simulink model "FOC"  (R2021b)
settings: Solver=ode45  StartTime=0.0  StopTime=1  MaxStep=1e-6  RelTol=1e-3
undefined symbols (not defined in the file): F, Flux, J, Ki_cd, Ki_cq, Ki_w, Kp_cd, Kp_cq, Kp_w, Ld, Lq, Np, Rs, Tf, Tmax, Tn, Ts, Udc, wn
libraries: slpidlib x3, spsUniversalBridgeLib x2, spsPermanentMagnetSynchronousMachineLib x1, spsSeriesRLCBranchLib x1, spsOnDelayLib x1, simulink x1, spsThreePhaseSourceLib x1, spsVoltageMeasurementLib x1, spspowerguiLib x1
settings Model: SimulationMode=accelerator  Creator=LFL  LastModifiedBy=Jiaxin Qian
settings SolverCC: AlgebraicLoopSolver=TrustRegion
settings DataIOCC: ReturnWorkspaceOutputs=off
settings DebuggingCC: SFMachineParentedDataDiag=warning  ArithmeticOperatorsInVariantConditions=warning
settings SFSimCC: SimUseLocalCustomCode=off  CustomCodeUndefinedFunction=UseInterfaceOnly
settings RTWCC: RTWUseLocalCustomCode=off

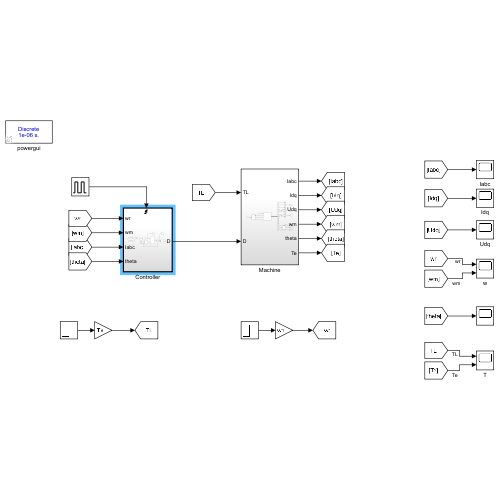
[thumbnail: Simulink's stored preview of the top-level diagram]
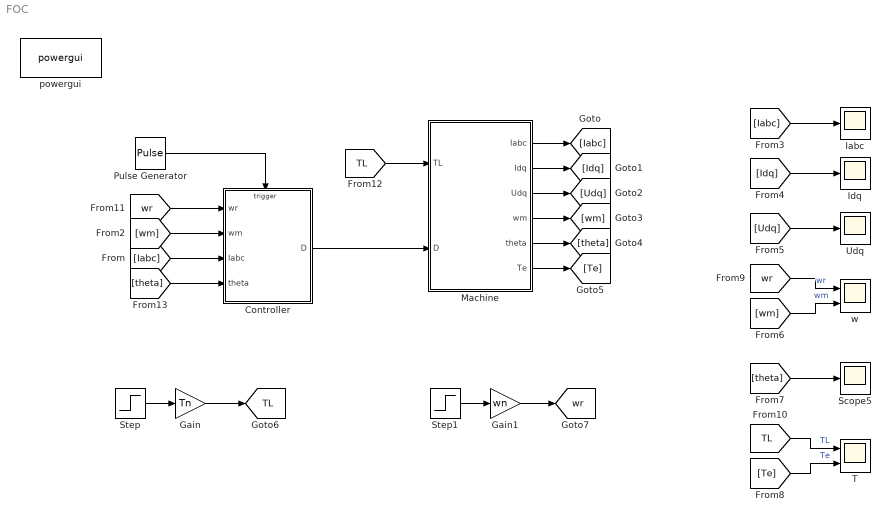
== system FOC ==
  Controller : Subsystem  TreatAsAtomicUnit=on
  Gain : Gain  Gain=Tn
  Gain1 : Gain  Gain=wn
  Iabc : Scope
  Idq : Scope
  Machine : Subsystem
  Pulse Generator : DiscretePulseGenerator  PulseType=Time based  Period=Ts  PulseWidth=50
  Scope5 : Scope
  Step : Step  Time=0.5  SampleTime=0
  Step1 : Step  Time=0  SampleTime=0
  T : Scope  NumInputPorts=2
  Udq : Scope
  powergui : spspowerguiLib/powergui  Priority=1  SimulationMode=Discrete  SampleTime=1e-6  frequency=60  Iterations=50  frequencyindice=0  Pbase=100e6  ErrMax=1e-4  UnitsV=kV  UnitsW=MW  buscounter=0  FunctionMessages=off  echomessages=off  EnableUseOfTLC=off  CurrentSourceSwitches=off  DisableSnubberDevices=off  DisableRonSwitches=off  DisableVfSwitches=off  DisplayEquations=off  AutomaticDiscreteSolvers=off  SolverType=Tustin/Backward Euler (TBE)  Interpol=off  ExternalGateDelay=off  methode=off  Ts=100  x0status=blocks  SPID=on  SwTol=0  HookPort=off  NonlinearTolerance=1e-4  nMaxIteration=100  ContinueOnMaxIteration=off  RestoreLinks=warning  ResistiveCurrentMeasurement=off  Frange=[0:2:500]  Ylog=off  Xlog=on  ShowGrid=off  save=off  variable=ZData  structure=0  ZoomFFT=off  StartTime=0.0  cycles=1  DisplayStyle=1  fundamental=60  FreqAxis=off  MaxFrequency=1000  frequencyindicesteady=1  RmsSteady=1  display=off
  w : Scope  NumInputPorts=2
  tag scope: TL=global, wr=global
  wires:
  Controller/1(D) -> Machine/2(D)
  Pulse Generator/1 -> Controller/Trigger
  Machine/1(Iabc) -> [Iabc]
  Machine/2(Idq) -> [Idq]
  Machine/3(Udq) -> [Udq]
  Machine/4(wm) -> [wm]
  Machine/5(theta) -> [theta]
  Machine/6(Te) -> [Te]
  [Iabc] -> Controller/3(Iabc)
  [wm] -> Controller/2(wm)
  [Iabc] -> Iabc/1
  [Udq] -> Udq/1
  [wm] -> w/2  "wm"
  [wr] -> w/1  "wr"
  [TL] -> T/1  "TL"
  [Te] -> T/2  "Te"
  [theta] -> Scope5/1
  [Idq] -> Idq/1
  [wr] -> Controller/1(wr)
  [TL] -> Machine/1(TL)
  [theta] -> Controller/4(theta)
  Step/1 -> Gain/1
  Gain/1 -> [TL]
  Step1/1 -> Gain1/1
  Gain1/1 -> [wr]

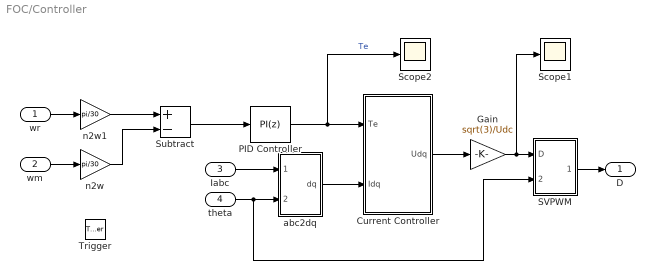
== system FOC/Controller ==
  wr : Inport
  wm : Inport  Port=2
  Iabc : Inport  Port=3
  theta : Inport  Port=4
  Trigger : TriggerPort  VariantControl=Variant
  Current Controller : Subsystem
  Gain : Gain  Gain=sqrt(3)/Udc
  PID Controller : slpidlib/PID Controller  Controller=PI  Form=Parallel  TimeDomain=Discrete-time  UseExternalTs=off  SampleTime=-1  IntegratorMethod=Forward Euler  FilterMethod=Forward Euler  ControllerParametersSource=internal  P=Kp_w  I=Ki_w  D=0  UseFilter=on  N=100  TunerSelectOption=Transfer Function Based (PID Tuner App)  InitialConditionSource=internal  InitialConditionForIntegrator=0  InitialConditionForFilter=0  DifferentiatorICPrevScaledInput=0  ExternalReset=none  TrackingMode=off  Kt=1  LimitOutput=on  SatLimitsSource=internal  UpperSaturationLimit=Tmax  LowerSaturationLimit=-Tmax  LinearizeAsGain=on  AntiWindupMode=clamping  Kb=1  POutMin=[]  POutMax=[]  IOutMin=[]  IOutMax=[]  DOutMin=[]  DOutMax=[]  NOutMin=[]  NOutMax=[]  SumOutMin=[]  SumOutMax=[]  SaturationOutMin=[]  SaturationOutMax=[]  PParamMin=[]  PParamMax=[]  IParamMin=[]  IParamMax=[]  DParamMin=[]  DParamMax=[]  NParamMin=[]  NParamMax=[]  KbParamMin=[]  KbParamMax=[]  KtParamMin=[]  KtParamMax=[]  KbOutMin=[]  KbOutMax=[]  KtOutMin=[]  KtOutMax=[]  IntegratorOutMin=[]  IntegratorOutMax=[]  FilterOutMin=[]  FilterOutMax=[]  SumI1OutMin=[]  SumI1OutMax=[]  SumI2OutMin=[]  SumI2OutMax=[]  SumI3OutMin=[]  SumI3OutMax=[]  SumI4OutMin=[]  SumI4OutMax=[]  SumDOutMin=[]  SumDOutMax=[]  DifferentiatorOutMin=[]  DifferentiatorOutMax=[]  FilterDiffOutCoefMin=[]  FilterDiffOutCoefMax=[]  ReciprocalOutMin=[]  ReciprocalOutMax=[]  SumDenOutMin=[]  SumDenOutMax=[]  SumNumOutMin=[]  SumNumOutMax=[]  DivideOutMin=[]  DivideOutMax=[]  UdiffTsProdOutMin=[]  UdiffTsProdOutMax=[]  NTsProdOutMin=[]  NTsProdOutMax=[]  UintegralTsProdOutMin=[]  UintegralTsProdOutMax=[]  UngainTsProdOutMin=[]  UngainTsProdOutMax=[]  IntegratorContinuousStateAttributes=''  IntegratorStateMustResolveToSignalObject=off  IntegratorRTWStateStorageClass=Auto  FilterContinuousStateAttributes=''  FilterStateMustResolveToSignalObject=off  FilterRTWStateStorageClass=Auto  ParallelPVariant=InternalParameters  IdealPVariant=Disabled  IVariant=InternalParameters  DVariant=Disabled  IntegratorVariant=Discrete  SatVariant=Enabled  AWVariant=DiscClampingParallel  PCopyVariant=Disabled  TRVariant=Disabled  FdbkBlocksVariant=Forward  IdealPFdbkVariant=Disabled  SatFdbkVariant=Disabled  DerivativeFilterVariant=Disabled  NVariant=Disabled  NCopyVariant=Disabled_SignalSpec  FilterICVariant=Disabled  IntegratorICVariant=InternalICs  ExternalResetVariant=Disabled  TRSumVariant=Passthrough  SumFdbkVariant=Disabled  SumVariant=Sum_PI  TsampFilterVariant=InternalTs  TsampNgainVariant=Passthrough  TsampIntegralVariant=Passthrough  ExternalSaturationOutDataTypeStr=Inherit: Same as second input
  SVPWM : Subsystem
  Scope1 : Scope
  Scope2 : Scope
  Subtract : Sum  Inputs=+-
  abc2dq : Subsystem
  n2w : Gain  Gain=pi/30
  n2w1 : Gain  Gain=pi/30
  D : Outport  VectorParamsAs1DForOutWhenUnconnected=off
  wires:
  wr/1 -> n2w1/1
  wm/1 -> n2w/1
  Subtract/1 -> PID Controller/1
  PID Controller/1 -> Scope2/1, Current Controller/1(Te)  "Te"
  Current Controller/1(Udq) -> Gain/1
  Gain/1 -> SVPWM/1(D), Scope1/1
  n2w/1 -> Subtract/2
  n2w1/1 -> Subtract/1
  abc2dq/1(dq) -> Current Controller/2(Idq)
  Iabc/1 -> abc2dq/1(abc)
  SVPWM/1(Dabc) -> D/1
  theta/1 -> SVPWM/2(theta), abc2dq/2(theta)

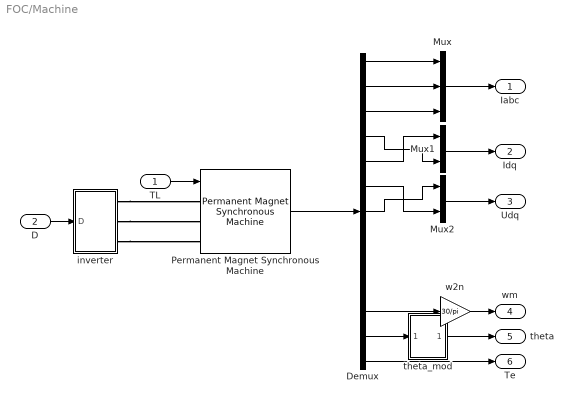
== system FOC/Machine ==
  TL : Inport
  D : Inport  Port=2
  Demux : Demux  Outputs=13
  Mux : Mux  Inputs=3
  Mux1 : Mux  Inputs=2
  Mux2 : Mux  Inputs=2
  Permanent Magnet Synchronous Machine : spsPermanentMagnetSynchronousMachineLib/Permanent Magnet Synchronous Machine  NbPhases=3  FluxDistribution=Sinusoidal  RotorType=Salient-pole  MechanicalLoad=Torque Tm  PresetModel=No  ShowDetailedParameters=on  MeasurementBus=off  Resistance=Rs  Inductance=8.5e-3  dqInductances=[Ld,Lq]  La=0.000395  MachineConstant=Flux linkage established by magnets (V.s)  Flux=Flux  VoltageCst=366.2061  TorqueCst=3.0285  Flat=120  Mechanical=[J F Np Tf]  PolePairs=4  InitialConditions=[0,0, 0,0]  InitialConditions5ph=[0 0 0 0 0 0]  RefAngle=Aligned with phase A axis (original Park)  IterativeDiscreteModel=Trapezoidal non iterative  TsBlock=-1  TsPowergui=0
  inverter : Subsystem
  theta_mod : Subsystem
  w2n : Gain  Gain=30/pi
  Iabc : Outport  VectorParamsAs1DForOutWhenUnconnected=off
  Idq : Outport  Port=2  VectorParamsAs1DForOutWhenUnconnected=off
  Udq : Outport  Port=3  VectorParamsAs1DForOutWhenUnconnected=off
  wm : Outport  Port=4  VectorParamsAs1DForOutWhenUnconnected=off
  theta : Outport  Port=5  VectorParamsAs1DForOutWhenUnconnected=off
  Te : Outport  Port=6  VectorParamsAs1DForOutWhenUnconnected=off
  wires:
  Permanent Magnet Synchronous Machine/1 -> Demux/1
  Demux/1 -> Mux/1
  Demux/2 -> Mux/2
  Demux/3 -> Mux/3
  Mux/1 -> Iabc/1
  Mux1/1 -> Idq/1
  Mux2/1 -> Udq/1
  Demux/11 -> w2n/1
  Demux/12 -> theta_mod/1(In1)
  Demux/13 -> Te/1
  TL/1 -> Permanent Magnet Synchronous Machine/1
  Demux/5 -> Mux1/1
  Demux/4 -> Mux1/2
  Demux/6 -> Mux2/2
  Demux/7 -> Mux2/1
  theta_mod/1(Out1) -> theta/1
  w2n/1 -> wm/1
  D/1 -> inverter/1(D)
  connections:
  inverter/RConn1 -- Permanent Magnet Synchronous Machine/LConn1
  inverter/RConn2 -- Permanent Magnet Synchronous Machine/LConn2
  inverter/RConn3 -- Permanent Magnet Synchronous Machine/LConn3

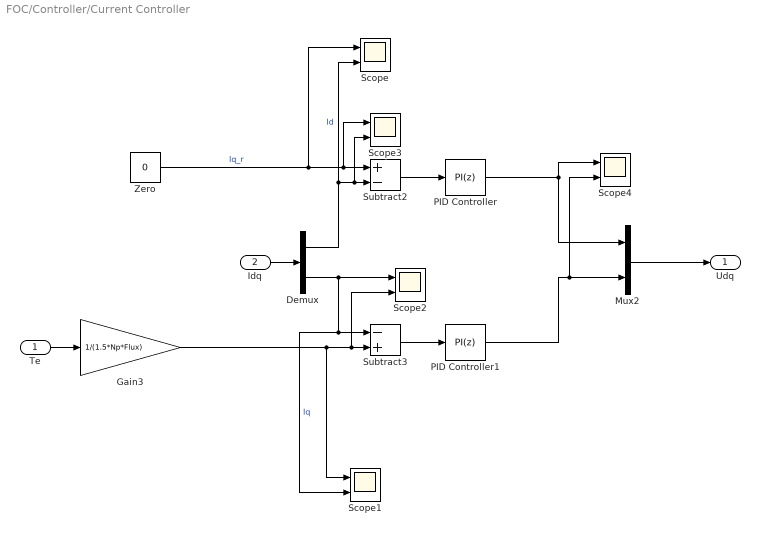
== system FOC/Controller/Current Controller ==
  Te : Inport
  Idq : Inport  Port=2
  Demux : Demux  Outputs=2
  Gain3 : Gain  Gain=1/(1.5*Np*Flux)
  Mux2 : Mux  Inputs=2
  PID Controller : slpidlib/PID Controller  Controller=PI  Form=Parallel  TimeDomain=Discrete-time  UseExternalTs=off  SampleTime=-1  IntegratorMethod=Forward Euler  FilterMethod=Forward Euler  ControllerParametersSource=internal  P=Kp_cd  I=Ki_cd  D=0  UseFilter=on  N=100  TunerSelectOption=Transfer Function Based (PID Tuner App)  InitialConditionSource=internal  InitialConditionForIntegrator=0  InitialConditionForFilter=0  DifferentiatorICPrevScaledInput=0  ExternalReset=none  TrackingMode=off  Kt=1  LimitOutput=off  SatLimitsSource=internal  UpperSaturationLimit=inf  LowerSaturationLimit=-inf  LinearizeAsGain=on  AntiWindupMode=none  Kb=1  POutMin=[]  POutMax=[]  IOutMin=[]  IOutMax=[]  DOutMin=[]  DOutMax=[]  NOutMin=[]  NOutMax=[]  SumOutMin=[]  SumOutMax=[]  SaturationOutMin=[]  SaturationOutMax=[]  PParamMin=[]  PParamMax=[]  IParamMin=[]  IParamMax=[]  DParamMin=[]  DParamMax=[]  NParamMin=[]  NParamMax=[]  KbParamMin=[]  KbParamMax=[]  KtParamMin=[]  KtParamMax=[]  KbOutMin=[]  KbOutMax=[]  KtOutMin=[]  KtOutMax=[]  IntegratorOutMin=[]  IntegratorOutMax=[]  FilterOutMin=[]  FilterOutMax=[]  SumI1OutMin=[]  SumI1OutMax=[]  SumI2OutMin=[]  SumI2OutMax=[]  SumI3OutMin=[]  SumI3OutMax=[]  SumI4OutMin=[]  SumI4OutMax=[]  SumDOutMin=[]  SumDOutMax=[]  DifferentiatorOutMin=[]  DifferentiatorOutMax=[]  FilterDiffOutCoefMin=[]  FilterDiffOutCoefMax=[]  ReciprocalOutMin=[]  ReciprocalOutMax=[]  SumDenOutMin=[]  SumDenOutMax=[]  SumNumOutMin=[]  SumNumOutMax=[]  DivideOutMin=[]  DivideOutMax=[]  UdiffTsProdOutMin=[]  UdiffTsProdOutMax=[]  NTsProdOutMin=[]  NTsProdOutMax=[]  UintegralTsProdOutMin=[]  UintegralTsProdOutMax=[]  UngainTsProdOutMin=[]  UngainTsProdOutMax=[]  IntegratorContinuousStateAttributes=''  IntegratorStateMustResolveToSignalObject=off  IntegratorRTWStateStorageClass=Auto  FilterContinuousStateAttributes=''  FilterStateMustResolveToSignalObject=off  FilterRTWStateStorageClass=Auto  ParallelPVariant=InternalParameters  IdealPVariant=Disabled  IVariant=InternalParameters  DVariant=Disabled  IntegratorVariant=Discrete  SatVariant=Disabled  AWVariant=Passthrough  PCopyVariant=Disabled  TRVariant=Disabled  FdbkBlocksVariant=Forward  IdealPFdbkVariant=Disabled  SatFdbkVariant=Disabled  DerivativeFilterVariant=Disabled  NVariant=Disabled  NCopyVariant=Disabled_SignalSpec  FilterICVariant=Disabled  IntegratorICVariant=InternalICs  ExternalResetVariant=Disabled  TRSumVariant=Passthrough  SumFdbkVariant=Disabled  SumVariant=Sum_PI  TsampFilterVariant=InternalTs  TsampNgainVariant=Passthrough  TsampIntegralVariant=Passthrough  ExternalSaturationOutDataTypeStr=Inherit: Same as second input
  PID Controller1 : slpidlib/PID Controller  Controller=PI  Form=Parallel  TimeDomain=Discrete-time  UseExternalTs=off  SampleTime=-1  IntegratorMethod=Forward Euler  FilterMethod=Forward Euler  ControllerParametersSource=internal  P=Kp_cq  I=Ki_cq  D=0  UseFilter=on  N=100  TunerSelectOption=Transfer Function Based (PID Tuner App)  InitialConditionSource=internal  InitialConditionForIntegrator=0  InitialConditionForFilter=0  DifferentiatorICPrevScaledInput=0  ExternalReset=none  TrackingMode=off  Kt=1  LimitOutput=off  SatLimitsSource=internal  UpperSaturationLimit=inf  LowerSaturationLimit=-inf  LinearizeAsGain=on  AntiWindupMode=none  Kb=1  POutMin=[]  POutMax=[]  IOutMin=[]  IOutMax=[]  DOutMin=[]  DOutMax=[]  NOutMin=[]  NOutMax=[]  SumOutMin=[]  SumOutMax=[]  SaturationOutMin=[]  SaturationOutMax=[]  PParamMin=[]  PParamMax=[]  IParamMin=[]  IParamMax=[]  DParamMin=[]  DParamMax=[]  NParamMin=[]  NParamMax=[]  KbParamMin=[]  KbParamMax=[]  KtParamMin=[]  KtParamMax=[]  KbOutMin=[]  KbOutMax=[]  KtOutMin=[]  KtOutMax=[]  IntegratorOutMin=[]  IntegratorOutMax=[]  FilterOutMin=[]  FilterOutMax=[]  SumI1OutMin=[]  SumI1OutMax=[]  SumI2OutMin=[]  SumI2OutMax=[]  SumI3OutMin=[]  SumI3OutMax=[]  SumI4OutMin=[]  SumI4OutMax=[]  SumDOutMin=[]  SumDOutMax=[]  DifferentiatorOutMin=[]  DifferentiatorOutMax=[]  FilterDiffOutCoefMin=[]  FilterDiffOutCoefMax=[]  ReciprocalOutMin=[]  ReciprocalOutMax=[]  SumDenOutMin=[]  SumDenOutMax=[]  SumNumOutMin=[]  SumNumOutMax=[]  DivideOutMin=[]  DivideOutMax=[]  UdiffTsProdOutMin=[]  UdiffTsProdOutMax=[]  NTsProdOutMin=[]  NTsProdOutMax=[]  UintegralTsProdOutMin=[]  UintegralTsProdOutMax=[]  UngainTsProdOutMin=[]  UngainTsProdOutMax=[]  IntegratorContinuousStateAttributes=''  IntegratorStateMustResolveToSignalObject=off  IntegratorRTWStateStorageClass=Auto  FilterContinuousStateAttributes=''  FilterStateMustResolveToSignalObject=off  FilterRTWStateStorageClass=Auto  ParallelPVariant=InternalParameters  IdealPVariant=Disabled  IVariant=InternalParameters  DVariant=Disabled  IntegratorVariant=Discrete  SatVariant=Disabled  AWVariant=Passthrough  PCopyVariant=Disabled  TRVariant=Disabled  FdbkBlocksVariant=Forward  IdealPFdbkVariant=Disabled  SatFdbkVariant=Disabled  DerivativeFilterVariant=Disabled  NVariant=Disabled  NCopyVariant=Disabled_SignalSpec  FilterICVariant=Disabled  IntegratorICVariant=InternalICs  ExternalResetVariant=Disabled  TRSumVariant=Passthrough  SumFdbkVariant=Disabled  SumVariant=Sum_PI  TsampFilterVariant=InternalTs  TsampNgainVariant=Passthrough  TsampIntegralVariant=Passthrough  ExternalSaturationOutDataTypeStr=Inherit: Same as second input
  Scope{,1..4} (5 alike) : Scope  NumInputPorts=2
  Subtract2 : Sum  Inputs=+-
  Subtract3 : Sum  Inputs=-+
  Zero : Constant  Value=0
  Udq : Outport  VectorParamsAs1DForOutWhenUnconnected=off
  wires:
  Mux2/1 -> Udq/1
  Idq/1 -> Demux/1
  Demux/1 -> Scope/2, Scope3/2, Subtract2/2  "Id"
  Demux/2 -> Scope2/1, Scope1/2, Subtract3/1  "Iq"
  Subtract2/1 -> PID Controller/1
  Subtract3/1 -> PID Controller1/1
  Zero/1 -> Scope3/1, Subtract2/1, Scope/1  "Iq_r"
  Te/1 -> Gain3/1
  Gain3/1 -> Scope2/2, Subtract3/2, Scope1/1
  PID Controller/1 -> Scope4/1, Mux2/1
  PID Controller1/1 -> Scope4/2, Mux2/2

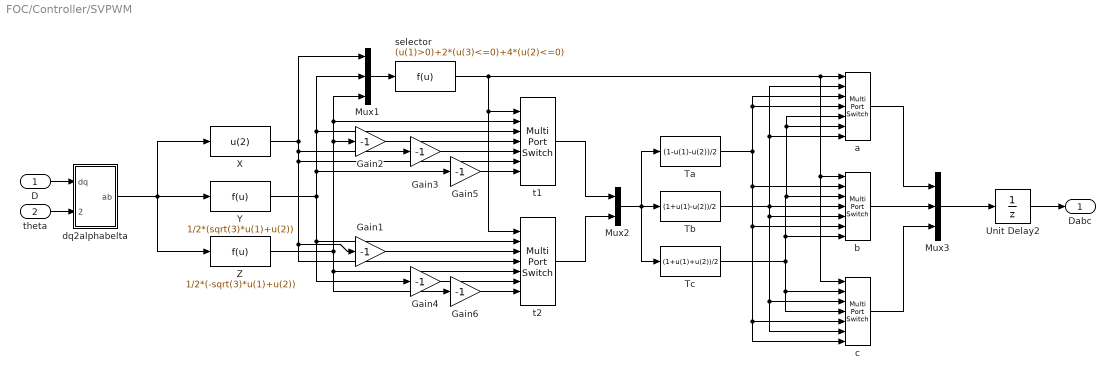
== system FOC/Controller/SVPWM ==
  D : Inport
  theta : Inport  Port=2
  Gain{1..6} (6 alike) : Gain  Gain=-1
  Mux1 : Mux  Inputs=3
  Mux2 : Mux  Inputs=2
  Mux3 : Mux  Inputs=3
  Ta : Fcn  Expr=(1-u(1)-u(2))/2
  Tb : Fcn  Expr=(1+u(1)-u(2))/2
  Tc : Fcn  Expr=(1+u(1)+u(2))/2
  Unit Delay2 : UnitDelay  SampleTime=-1  HasFrameUpgradeWarning=on
  X : Fcn  Expr=u(2)
  Y : Fcn  Expr=1/2*(sqrt(3)*u(1)+u(2))
  Z : Fcn  Expr=1/2*(-sqrt(3)*u(1)+u(2))
  a : MultiPortSwitch  Inputs=6
  b : MultiPortSwitch  Inputs=6
  c : MultiPortSwitch  Inputs=6
  dq2alphabelta : Subsystem
  selector : Fcn  Expr=(u(1)>0)+2*(u(3)<=0)+4*(u(2)<=0)
  t1 : MultiPortSwitch  Inputs=6
  t2 : MultiPortSwitch  Inputs=6
  Dabc : Outport  VectorParamsAs1DForOutWhenUnconnected=off
  wires:
  theta/1 -> dq2alphabelta/2(theta)
  X/1 -> Gain3/1, t1/6, Gain1/1, t2/4, Mux1/1
  Y/1 -> Gain5/1, t1/3, Mux1/2, Gain4/1, t2/2
  Z/1 -> Gain6/1, t2/5, Gain2/1, t1/2, Mux1/3
  Mux1/1 -> selector/1
  selector/1 -> c/1, b/1, a/1, t2/1, t1/1
  Gain1/1 -> t2/3
  Gain2/1 -> t1/4
  Gain3/1 -> t1/5
  Gain4/1 -> t2/6
  Gain5/1 -> t1/7
  Gain6/1 -> t2/7
  t1/1 -> Mux2/1
  t2/1 -> Mux2/2
  Mux2/1 -> Tc/1, Ta/1, Tb/1
  Tb/1 -> b/4, b/5, c/6, c/3, a/7, a/2
  Ta/1 -> a/4, a/3, b/6, c/7, c/5, b/2
  Tc/1 -> b/7, a/6, a/5, b/3, c/2, c/4
  b/1 -> Mux3/2
  a/1 -> Mux3/1
  c/1 -> Mux3/3
  dq2alphabelta/1(ab) -> Z/1, X/1, Y/1
  Unit Delay2/1 -> Dabc/1
  Mux3/1 -> Unit Delay2/1
  D/1 -> dq2alphabelta/1(dq)

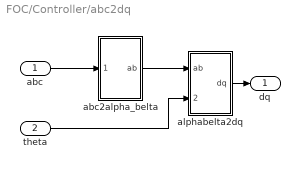
== system FOC/Controller/abc2dq ==
  abc : Inport
  theta : Inport  Port=2
  abc2alpha_belta : Subsystem
  alphabelta2dq : Subsystem
  dq : Outport  VectorParamsAs1DForOutWhenUnconnected=off
  wires:
  abc/1 -> abc2alpha_belta/1(abc)
  abc2alpha_belta/1(ab) -> alphabelta2dq/1(ab)
  alphabelta2dq/1(dq) -> dq/1
  theta/1 -> alphabelta2dq/2(theta)

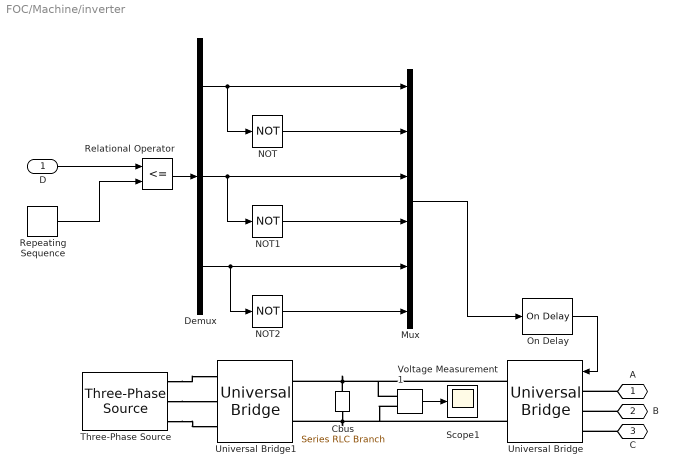
== system FOC/Machine/inverter ==
  D : Inport
  Cbus : spsSeriesRLCBranchLib/Series RLC Branch  LConnTagsString=__new0  RConnTagsString=__new0  BranchType=C  Resistance=1  Inductance=1e-3  SetiL0=off  InitialCurrent=0  Capacitance=4e-3  Setx0=on  InitialVoltage=0  Measurements=None
  Demux : Demux  Outputs=3
  Mux : Mux  Inputs=6
  NOT : Logic  Operator=NOT  IconShape=distinctive  AllPortsSameDT=off  OutDataTypeStr=boolean
  NOT1 : Logic  Operator=NOT  IconShape=distinctive  AllPortsSameDT=off  OutDataTypeStr=boolean
  NOT2 : Logic  Operator=NOT  IconShape=distinctive  AllPortsSameDT=off  OutDataTypeStr=boolean
  On Delay : spsOnDelayLib/On Delay  DelayType=On delay  delay=Deadtime  ic=0  Ts=0
      settings: SourceProductBaseCode=PS
  Relational Operator : RelationalOperator  Operator=<=  OutDataTypeStr=boolean  RndMeth=Simplest
  Repeating Sequence : simulink/Sources/Repeating Sequence  rep_seq_t=[0 Ts/2 Ts]  rep_seq_y=[0 1 0]
  Scope1 : Scope
  Three-Phase Source : spsThreePhaseSourceLib/Three-Phase Source  InternalConnection=Yg  VoltagePhases=off  Voltage=380  PhaseAngle=0  Voltage_phases=[25e3 25e3 25e3]/sqrt(3)  PhaseAngles_phases=[0 -120 +120]  Frequency=50  NonIdealSource=off  SpecifyImpedance=off  Resistance=0.8929  Inductance=16.58e-3  ShortCircuitLevel=100e6  BaseVoltage=25e3  XRratio=7  BusType=swing  Pref=10e3  Qref=0  Prefabc=[10e3, 10e3, 10e3]  Qrefabc=[0, 0, 0]  Qmin=-inf  Qmax=inf
  Universal Bridge : spsUniversalBridgeLib/Universal Bridge  Arms=3  SnubberResistance=1e5  SnubberCapacitance=inf  Device=MOSFET / Diodes  Ron=1e-3  Lon=0  ForwardVoltages="[  0  0  ]"  ForwardVoltage=0  GTOparameters=[ 10e-6 , 20e-6 ]  IGBTparameters=[ 1e-6 , 2e-6 ]  Measurements=None  Measurements_2=None  converterType=Rectifier
  Universal Bridge1 : spsUniversalBridgeLib/Universal Bridge  Arms=3  SnubberResistance=1e5  SnubberCapacitance=inf  Device=Diodes  Ron=1e-3  Lon=0  ForwardVoltages="[  0  0  ]"  ForwardVoltage=0  GTOparameters=[ 10e-6 , 20e-6 ]  IGBTparameters=[ 1e-6 , 2e-6 ]  Measurements=None  Measurements_2=None  converterType=Rectifier
  Voltage Measurement1 : spsVoltageMeasurementLib/Voltage Measurement  PhasorSimulation=off  OutputType=Complex  PSBequivalent=0
  A : PMIOPort  Side=Right
  B : PMIOPort  Port=2  Side=Right
  C : PMIOPort  Port=3  Side=Right
  wires:
  On Delay/1 -> Universal Bridge/1
  NOT1/1 -> Mux/4
  NOT/1 -> Mux/2
  Demux/1 -> Mux/1, NOT/1
  Demux/3 -> NOT2/1, Mux/5
  Demux/2 -> NOT1/1, Mux/3
  NOT2/1 -> Mux/6
  Relational Operator/1 -> Demux/1
  D/1 -> Relational Operator/1
  Mux/1 -> On Delay/1
  Repeating Sequence/1 -> Relational Operator/2
  Voltage Measurement1/1 -> Scope1/1
  connections:
  A/RConn1 -- Universal Bridge/LConn1
  B/RConn1 -- Universal Bridge/LConn2
  C/RConn1 -- Universal Bridge/LConn3
  Cbus/LConn1 -- Universal Bridge1/RConn1 -- Universal Bridge/RConn1 -- Voltage Measurement1/LConn1
  Cbus/RConn1 -- Universal Bridge1/RConn2 -- Universal Bridge/RConn2 -- Voltage Measurement1/LConn2
  Three-Phase Source/RConn2 -- Universal Bridge1/LConn2
  Three-Phase Source/RConn1 -- Universal Bridge1/LConn1
  Three-Phase Source/RConn3 -- Universal Bridge1/LConn3

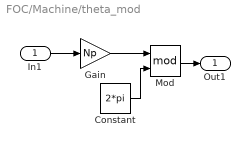
== system FOC/Machine/theta_mod ==
  In1 : Inport
  Constant : Constant  Value=2*pi
  Gain : Gain  Gain=Np
  Mod : Math  Operator=mod  SignedPower=on  SaturateOnIntegerOverflow=on
  Out1 : Outport  VectorParamsAs1DForOutWhenUnconnected=off
  wires:
  Mod/1 -> Out1/1
  Constant/1 -> Mod/2
  In1/1 -> Gain/1
  Gain/1 -> Mod/1

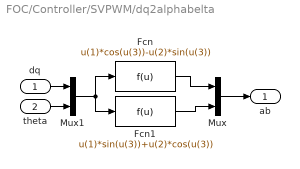
== system FOC/Controller/SVPWM/dq2alphabelta ==
  dq : Inport
  theta : Inport  Port=2
  Fcn : Fcn  Expr=u(1)*cos(u(3))-u(2)*sin(u(3))
  Fcn1 : Fcn  Expr=u(1)*sin(u(3))+u(2)*cos(u(3))
  Mux : Mux  Inputs=2
  Mux1 : Mux  Inputs=2
  ab : Outport  VectorParamsAs1DForOutWhenUnconnected=off
  wires:
  Mux/1 -> ab/1
  dq/1 -> Mux1/1
  theta/1 -> Mux1/2
  Mux1/1 -> Fcn/1, Fcn1/1
  Fcn/1 -> Mux/1
  Fcn1/1 -> Mux/2

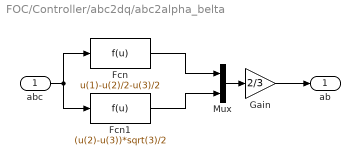
== system FOC/Controller/abc2dq/abc2alpha_belta ==
  abc : Inport
  Fcn : Fcn  Expr=u(1)-u(2)/2-u(3)/2
  Fcn1 : Fcn  Expr=(u(2)-u(3))*sqrt(3)/2
  Gain : Gain  Gain=2/3
  Mux : Mux  Inputs=2
  ab : Outport  VectorParamsAs1DForOutWhenUnconnected=off
  wires:
  abc/1 -> Fcn/1, Fcn1/1
  Fcn/1 -> Mux/1
  Fcn1/1 -> Mux/2
  Mux/1 -> Gain/1
  Gain/1 -> ab/1

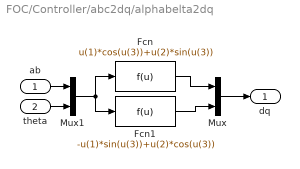
== system FOC/Controller/abc2dq/alphabelta2dq ==
  ab : Inport
  theta : Inport  Port=2
  Fcn : Fcn  Expr=u(1)*cos(u(3))+u(2)*sin(u(3))
  Fcn1 : Fcn  Expr=-u(1)*sin(u(3))+u(2)*cos(u(3))
  Mux : Mux  Inputs=2
  Mux1 : Mux  Inputs=2
  dq : Outport  VectorParamsAs1DForOutWhenUnconnected=off
  wires:
  Mux/1 -> dq/1
  ab/1 -> Mux1/1
  theta/1 -> Mux1/2
  Mux1/1 -> Fcn/1, Fcn1/1
  Fcn/1 -> Mux/1
  Fcn1/1 -> Mux/2
